simulink model "uz_ResonantController_2022a"  (R2022a)
settings: Solver=FixedStepDiscrete  StartTime=0.0  StopTime=0.01  RelTol=1e-3  EnableMultiTasking=on
PreLoadFcn:
  | uz_setCodegenPaths
model workspace (MATLAB code in the model file):
  | cmdLim = Simulink.Parameter;
  | cmdLim.Value = 15;
  | cmdLim.Description = 'Limit for controlling the maximum surface command angle.';
  | cmdLim.Min = 0;
  | cmdLim.Max = 90;
  | cmdLim.DocUnits = 'deg';
  | 
  | dispGain = Simulink.Parameter;
  | dispGain.Value = 0.75;
  | dispGain.Description = 'Gain applied to the displacement error.';
  | dispGain.Min = 0;
  | dispGain.Max = [];
  | dispGain.DocUnits = 'deg/sec/deg';
  | 
  | dispLim = Simulink.Parameter;
  | dispLim.Value = 30;
  | dispLim.Description = 'Limit for controlling the maximum commanded angle.';
  | dispLim.Min = 0;
  | dispLim.Max = 180;
  | dispLim.DocUnits = 'deg';
  | 
  | intGain = Simulink.Parameter;
  | intGain.Value = 0.5;
  | intGain.Description = 'Gain applied to the integral error.';
  | intGain.Min = 0;
  | intGain.Max = [];
  | intGain.DocUnits = 'deg/sec/deg/sec';
  | 
  | intLim = Simulink.Parameter;
  | intLim.Value = 5;
  | intLim.Description = 'Limit for controlling the maximum commanded angle.';
  | intLim.Min = 0;
  | intLim.Max = 90;
  | intLim.DocUnits = 'deg';
  | 
  | rateGain = Simulink.Parameter;
  | rateGain.Value = 2;
  | rateGain.Description = 'Gain applied to the rate error.';
  | rateGain.Min = 0;
  | rateGain.Max = [];
  | rateGain.DocUnits = 'deg/deg/sec';
  | 
  | rateLim = Simulink.Parameter;
  | rateLim.Value = 6;
  | rateLim.Description = 'Limit for controlling the maximum commanded angle.';
  | rateLim.Min = 0;
  | rateLim.Max = 180;
  | rateLim.DocUnits = 'deg/sec';
  | 
  | hdgGain = Simulink.Parameter;
  | hdgGain.Value = 0.015;
undefined symbols (not defined in the file or in its folder): DiscIntNeverNeededParam, f_c
libraries: simulink x1
settings Model: RequirementInfo={} %GIDa_fe9045fd_0412_4b6e_8206_617cc20e6fde  FPTRunName=Active  Creator=ts  LastModifiedBy=Josef Knoblach
settings SolverCC: AlgebraicLoopSolver=TrustRegion  PositivePriorityOrder=on  AutoInsertRateTranBlk=on
settings DataIOCC: SaveOutput=off  SignalLogging=off  DSMLogging=off  SaveTime=off
settings OptimizationCC: DefaultParameterBehavior=Inlined  UseDivisionForNetSlopeComputation=on  GainParamInheritBuiltInType=on  UseFloatMulNetSlope=on  UseSpecifiedMinMax=on  InlineInvariantSignals=on  PassReuseOutputArgsAs=Individual arguments  NoFixptDivByZeroProtection=on  EfficientFloat2IntCast=on  LifeSpan=1  MaxStackSize=64  OptimizeBlockOrder=speed  DifferentSizesBufferReuse=on  EfficientTunableParamExpr=on
settings DebuggingCC: UnconnectedInputMsg=warning  UnconnectedOutputMsg=warning  UnconnectedLineMsg=warning  AllowSymbolicDim=off  SFUnexpectedBacktrackingDiag=warning  SFNoUnconditionalDefaultTransitionDiag=warning  SFExecutionAtInitializationDiag=none  SFMachineParentedDataDiag=warning  ArithmeticOperatorsInVariantConditions=warning
settings HardwareCC: ProdBitPerPointer=32  ProdBitPerSizeT=32  ProdBitPerPtrDiffT=32  ProdLargestAtomicInteger=Long  ProdLargestAtomicFloat=Double  ProdWordSize=32  ProdLongLongMode=on  ProdHWDeviceType=ARM Compatible->ARM Cortex-R  HardwareBoardFeatureSet=SoCBlockset
settings SFSimCC: MATLABDynamicMemAlloc=off
settings RTWCC: SystemTargetFile=ert.tlc  GenCodeOnly=on  TemplateMakefile=ert_default_tmf  GenerateReport=on  BuildConfiguration=Faster Runs  IncludeHyperlinkInReport=on  GenerateCodeMetricsReport=on  CheckMdlBeforeBuild=Warning  DLArmComputeVersion=19.05
settings CodeAppCC: ForceParamTrailComments=on  IgnoreCustomStorageClasses=off  OperatorAnnotations=on  SimulinkDataObjDesc=on  SFDataObjDesc=on  MATLABFcnDesc=on  InsertBlockDesc=on  StateflowObjectComments=on  MATLABSourceComments=on  EnableCustomComments=on  ReqsInCode=on
settings ERTTargetCC: TargetLangStandard=C99 (ISO)  CodeReplacementLibrary=GNU C99 extensions  MultiwordLength=2048  IncludeMdlTerminateFcn=off  CombineSignalStateStructs=on  SuppressErrorStatus=on  IncludeFileDelimiter=UseQuote  SupportAbsoluteTime=off  CodeInterfacePackaging=Reusable function  SupportNonFinite=off  RemoveResetFunc=off  InlinedParameterPlacement=NonHierarchical  MultiInstanceErrorCode=Warning  RootIOFormat=Part of model data structure  ERTCustomFileTemplate=example_file_process.tlc  GlobalDataDefinition=InSourceFile  GlobalDataReference=InSourceFile  ERTFilePackagingFormat=CompactWithDataFile
settings ConfigComp: CovScope=ReferencedModels  CovSaveName=covdata_rollAP  CovMetricSettings=dcmtrwe  CovHTMLOptions=-sRT=1 -aTS=1 -bRG=1 -bTC=1 -hTR=1 -nFC=0 -scm=1 -bcm=1 -xEv=0  CovSaveCumulativeToWorkspaceVar=on  CovSaveSingleToWorkspaceVar=on  CovCumulativeVarName=covCumulativeData_rollAP  CovReportOnPause=off  CovExternalEMLEnable=off  CovSFcnEnable=off

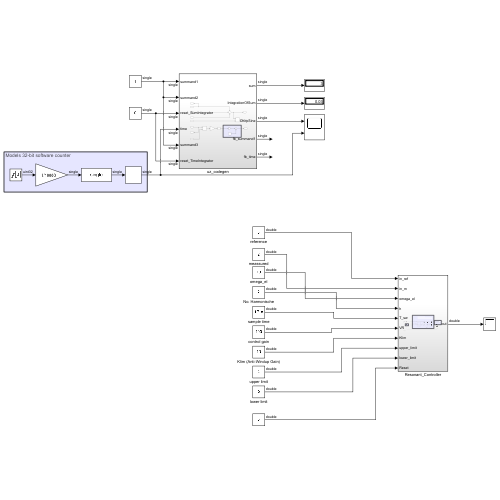
[thumbnail: Simulink's stored preview of the top-level diagram]
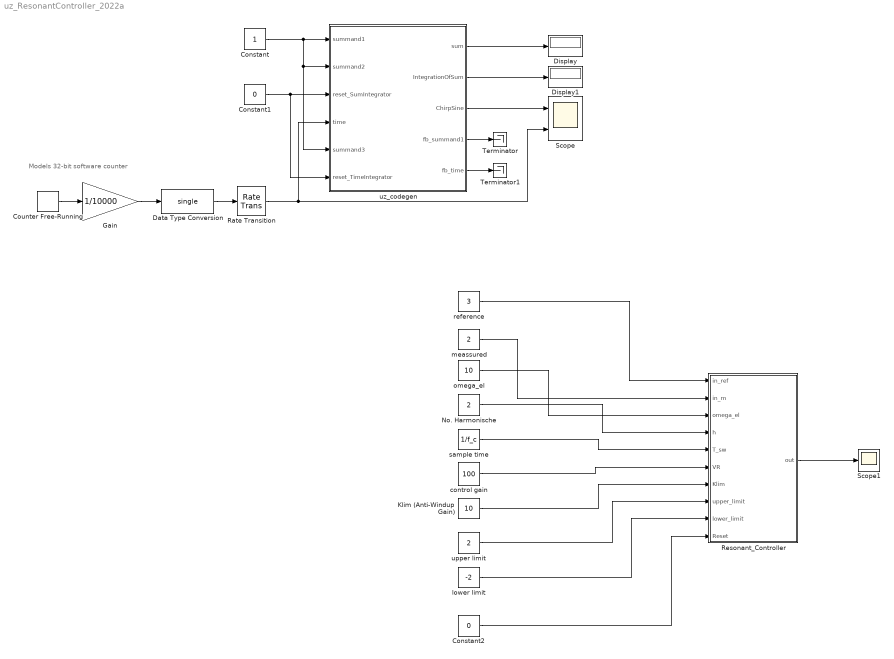
== system uz_ResonantController_2022a ==
  note: Models 32-bit software counter
  Constant : Constant  OutDataTypeStr=single  SampleTime=1/10000
  Constant1 : Constant  Value=0  OutDataTypeStr=single  SampleTime=1/10000
  Constant2 : Constant  Value=0
  Counter Free-Running : simulink/Sources/Counter Free-Running  NumBits=32  tsamp=1/10000
  Data Type Conversion : DataTypeConversion  OutDataTypeStr=single  SaturateOnIntegerOverflow=off  RndMeth=Floor
  Display : Display
  Display1 : Display
  Gain : Gain  Gain=1/10000  OutDataTypeStr=single
  Klim (Anti-Windup Gain) : Constant  Value=10
  No. Harmonische : Constant  Value=2
  Rate Transition : RateTransition  OutPortSampleTime=1/10000
  Resonant_Controller : Subsystem
  Scope : Scope  NumInputPorts=2
  Scope1 : Scope
  Terminator : Terminator
  Terminator1 : Terminator
  control gain : Constant  Value=100
  lower limit : Constant  Value=-2
  meassured : Constant  Value=2
  omega_el : Constant  Value=10
  reference : Constant  Value=3
  sample time : Constant  Value=1/f_c
  upper limit : Constant  Value=2
  uz_codegen : Subsystem
  wires:
  uz_codegen/1(sum) -> Display/1
  Constant/1 -> uz_codegen/5(summand3), uz_codegen/2(summand2), uz_codegen/1(summand1)
  uz_codegen/2(IntegrationOfSum) -> Display1/1
  uz_codegen/3(ChirpSine) -> Scope/1
  Constant1/1 -> uz_codegen/6(reset_TimeIntegrator), uz_codegen/3(reset_SumIntegrator)
  Gain/1 -> Data Type Conversion/1
  Rate Transition/1 -> uz_codegen/4(time), Scope/2
  Data Type Conversion/1 -> Rate Transition/1
  uz_codegen/4(fb_summand1) -> Terminator/1
  Counter Free-Running/1 -> Gain/1
  uz_codegen/5(fb_time) -> Terminator1/1
  sample time/1 -> Resonant_Controller/5(T_sw)
  No. Harmonische/1 -> Resonant_Controller/4(h)
  reference/1 -> Resonant_Controller/1(in_ref)
  meassured/1 -> Resonant_Controller/2(in_m)
  control gain/1 -> Resonant_Controller/6(VR)
  omega_el/1 -> Resonant_Controller/3(omega_el)
  Resonant_Controller/1(out) -> Scope1/1
  Klim (Anti-Windup Gain)/1 -> Resonant_Controller/7(Klim)
  upper limit/1 -> Resonant_Controller/8(upper_limit)
  lower limit/1 -> Resonant_Controller/9(lower_limit)
  Constant2/1 -> Resonant_Controller/10(Reset)

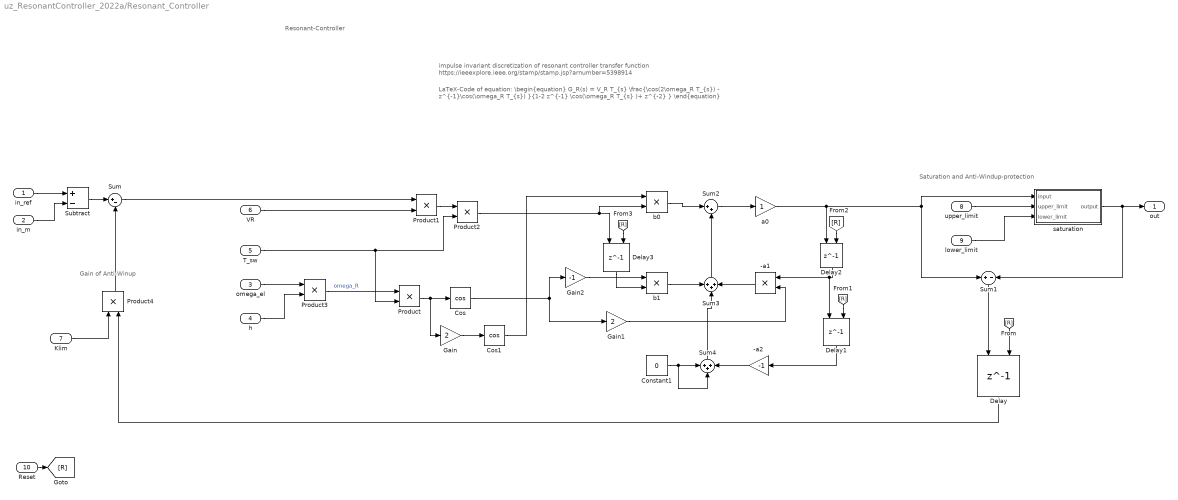
== system uz_ResonantController_2022a/Resonant_Controller ==
  note: Gain of Anti-Winup
  note: Saturation and Anti-Windup-protection
  note: Resonant-Controller
  note: impulse invariant discretization of resonant controller transfer function
      | https://ieeexplore.ieee.org/stamp/stamp.jsp?arnumber=5398914
  note: LaTeX-Code of equation:
      | \begin{equation}
      | 	G_R(s) = V_R T_{s} \frac{\cos(2\omega_R T_{s}) - z^{-1}\cos(\omega_R T_{s}) }{1-2 z^{-1} \cos(\omega_R T_{s} )+ z^{-2} }
      | \end{equation}
  in_ref : Inport
  in_m : Inport  Port=2
  omega_el : Inport  Port=3
  h : Inport  Port=4
  T_sw : Inport  Port=5
  VR : Inport  Port=6
  Klim : Inport  Port=7
  upper_limit : Inport  Port=8
  lower_limit : Inport  Port=9
  Reset : Inport  Port=10
  -a1 : Product
  -a2 : Gain  Gain=-1
  Constant1 : Constant  Value=0
  Cos : Trigonometry  Operator=cos
  Cos1 : Trigonometry  Operator=cos
  Delay{,1..3} (4 alike) : Delay  DelayLength=1  InitialCondition=0  ExternalReset=Level hold  SampleTime=1/f_c
      settings: InputPortMap=u0,r5
  Gain : Gain  Gain=2
  Gain1 : Gain  Gain=2
  Gain2 : Gain  Gain=-1
  Product{,1..4} (5 alike) : Product
  Subtract : Sum  Inputs=+-
  Sum : Sum  Inputs=|+-
  Sum1 : Sum  Inputs=+|-
  Sum2 : Sum  Inputs=|++
  Sum3 : Sum  Inputs=+++
  Sum4 : Sum  Inputs=+++
  a0 : Gain
  b0 : Product
  b1 : Product
  saturation : MATLAB Function  TreatAsAtomicUnit=on
  out : Outport
  wires:
  Cos/1 -> Gain1/1, Gain2/1
  T_sw/1 -> Product/2, Product2/2
  Product/1 -> Gain/1, Cos/1
  Gain/1 -> Cos1/1
  Sum4/1 -> Sum3/2
  b1/1 -> Sum3/1
  -a1/1 -> Sum3/3
  Delay2/1 -> -a1/1, Delay1/1
  Delay1/1 -> -a2/1
  -a2/1 -> Sum4/3
  Delay3/1 -> b1/2
  b0/1 -> Sum2/1
  Sum3/1 -> Sum2/2
  Sum2/1 -> a0/1
  a0/1 -> saturation/1(input), Sum1/1, Delay2/1
  Constant1/1 -> Sum4/1, Sum4/2
  Gain1/1 -> -a1/2
  Product1/1 -> Product2/1
  Product2/1 -> Delay3/1, b0/2
  omega_el/1 -> Product3/1
  Product3/1 -> Product/1  "omega_R"
  h/1 -> Product3/2
  Cos1/1 -> b0/1
  Gain2/1 -> b1/1
  VR/1 -> Product1/2
  in_ref/1 -> Subtract/1
  in_m/1 -> Subtract/2
  Subtract/1 -> Sum/1
  Sum/1 -> Product1/1
  Product4/1 -> Sum/2
  Klim/1 -> Product4/1
  Sum1/1 -> Delay/1
  saturation/1(output) -> Sum1/2, out/1
  upper_limit/1 -> saturation/2(upper_limit)
  lower_limit/1 -> saturation/3(lower_limit)
  Delay/1 -> Product4/2
  Reset/1 -> [R]
  [R] -> Delay/2
  [R] -> Delay1/2
  [R] -> Delay2/2
  [R] -> Delay3/2

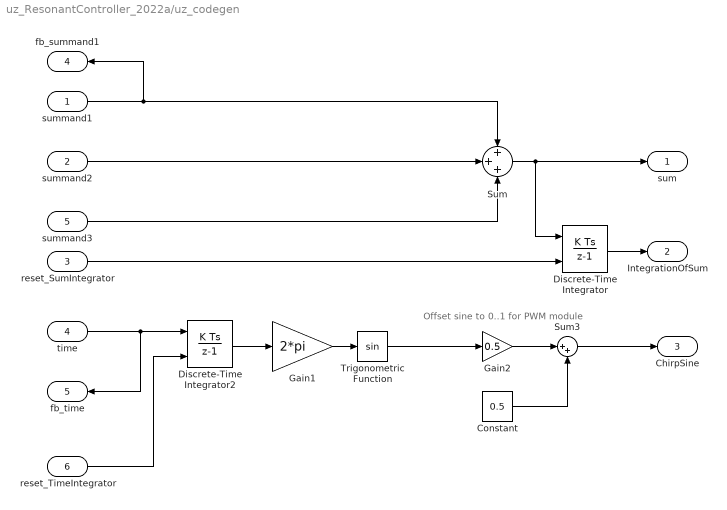
== system uz_ResonantController_2022a/uz_codegen ==
  note: Offset sine to 0..1 for PWM module
  summand1 : Inport  OutDataTypeStr=single
  summand2 : Inport  Port=2  OutDataTypeStr=single
  reset_SumIntegrator : Inport  Port=3  OutDataTypeStr=single
  time : Inport  Port=4  OutDataTypeStr=single
  summand3 : Inport  Port=5  OutDataTypeStr=single
  reset_TimeIntegrator : Inport  Port=6  OutDataTypeStr=single
  Constant : Constant  Value=0.5  OutDataTypeStr=single
  Discrete-Time Integrator : DiscreteIntegrator  ExternalReset=level  SampleTime=-1  UpperSaturationLimit=1000  LowerSaturationLimit=-1000  ICPrevOutput=DiscIntNeverNeededParam  ICPrevScaledInput=DiscIntNeverNeededParam
  Discrete-Time Integrator2 : DiscreteIntegrator  ExternalReset=level  SampleTime=-1  UpperSaturationLimit=1000  LowerSaturationLimit=-1000  ICPrevOutput=DiscIntNeverNeededParam  ICPrevScaledInput=DiscIntNeverNeededParam
  Gain1 : Gain  Gain=2*pi
  Gain2 : Gain  Gain=0.5
  Sum : Sum  Inputs=+++  InputSameDT=on  OutDataTypeStr=Inherit: Same as first input
  Sum3 : Sum  Inputs=|++
  Trigonometric Function : Trigonometry
  sum : Outport  VectorParamsAs1DForOutWhenUnconnected=off
  IntegrationOfSum : Outport  Port=2  VectorParamsAs1DForOutWhenUnconnected=off
  ChirpSine : Outport  Port=3  VectorParamsAs1DForOutWhenUnconnected=off
  fb_summand1 : Outport  Port=4  VectorParamsAs1DForOutWhenUnconnected=off
  fb_time : Outport  Port=5  VectorParamsAs1DForOutWhenUnconnected=off
  wires:
  summand1/1 -> Sum/1, fb_summand1/1
  summand2/1 -> Sum/2
  Sum/1 -> sum/1, Discrete-Time Integrator/1
  Discrete-Time Integrator/1 -> IntegrationOfSum/1
  Gain1/1 -> Trigonometric Function/1
  Trigonometric Function/1 -> Gain2/1
  Gain2/1 -> Sum3/1
  Constant/1 -> Sum3/2
  Sum3/1 -> ChirpSine/1
  time/1 -> fb_time/1, Discrete-Time Integrator2/1
  reset_SumIntegrator/1 -> Discrete-Time Integrator/2
  Discrete-Time Integrator2/1 -> Gain1/1
  summand3/1 -> Sum/3
  reset_TimeIntegrator/1 -> Discrete-Time Integrator2/2

== matlab function uz_ResonantController_2022a/Resonant_Controller/saturation ==
  data: input input; output output; upper_limit input; lower_limit input
function output = fcn(input, upper_limit, lower_limit)

output = input;

if (input > upper_limit)
    output = upper_limit;
end

if (input < lower_limit)
    output = lower_limit;
end
